simulink model "todayIntegrirAndDifferenc"  (R2016a)
settings: Solver=VariableStepAuto  StartTime=0.0  StopTime=10.0  RelTol=1e-3
settings Model: Creator=Ivan Varabei  LastModifiedBy=Ivan Varabei

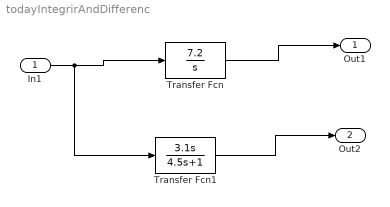
== system todayIntegrirAndDifferenc ==
  In1 : Inport
  Transfer Fcn : TransferFcn  Numerator=[7.2]  Denominator=[1 0]
  Transfer Fcn1 : TransferFcn  Numerator=[3.1 0]  Denominator=[4.5 1]
  Out1 : Outport
  Out2 : Outport  Port=2
  wires:
  Transfer Fcn/1 -> Out1/1
  Transfer Fcn1/1 -> Out2/1
  In1/1 -> Transfer Fcn1/1, Transfer Fcn/1
